simulink model "OMSv1_4"  (Simulink 7.0)
settings: Solver=ode4  SolverMode=SingleTasking  StartTime=0.0  StopTime=4  FixedStep=0.001  MaxStep=0.001  RelTol=1e-3  AbsTol=1e-3
undefined symbols (not defined in the file): alexlaw, bs_onoff, bs_scale, bsfsacrit, bsfsvcrit, cnsgain, fs_onoff, fs_scale, fsdelaycalc, ltdrk, mdlparamlist, phasicgain, pmcgain, pmctau2, pmctau3, saccsw, spgain, tonicgain, tvrD, tvrN
(part 5 of 10)

== system OMSv1_4/OMS v1.4  12/31/07/IM CN-LMLN/BS/FS Logic/BS Enable1/BS Timing ==
  note: (FF init state: Q=0)
  note: * Leading Edge of input ENABLEs output
  note: Operation:
  note: *BS Enabling is initially DISABLED
  note: * Output of TIMER circuit DISABLES output
  note: BS Timing
  From  <= [cmpr] : Inport  OutDataType=sfix(16)  OutScaling=2^0
  timer dur : Inport  Orientation=up  Port=2  OutDataType=sfix(16)  OutScaling=2^0
  Latch1 : Subsystem  mask(Latch){@1=0}
      mask prompts: @1 "Initial State for Output "Q":"
      mask help: Latch
      mask init:
      | ini=(@1~=0);
      mask Help: Latches the S input.  When S (set) is one, the Q output  becomes one.  The output remains one until the R (reset) input becomes one, forcing the output to zero.  If both R and S are one, the latch will be in an undefined state.
      mask Display: disp('S   Q\n\nR  !Q')
  Terminator : Terminator
  event timer2 : Subsystem
      mask Display: disp('Event\nTimer2')
  leading edge detect : Subsystem
      mask Display: disp('Leading\nEdge Det')
  "[bsenab]" : Outport  OutDataType=sfix(16)  OutScaling=2^0  InitialOutput=0
  wires:
  From  <= [cmpr]/1 -> leading edge detect/1(in_1), event timer2/1(_PG)
  leading edge detect/1(out_1) -> Latch1/1(in_1)
  event timer2/1(out_1) -> Latch1/2(in_2)
  Latch1/1(out_1) -> "[bsenab]"/1
  timer dur/1 -> event timer2/2(_timer value (port))
  Latch1/2(out_2) -> Terminator/1

== system OMSv1_4/OMS v1.4  12/31/07/IM CN-LMLN/BS/FS Logic/FS Enable/FS Timing ==
  note: FS Timing
  note: * Output of TIMER circuit DISABLES output
  note: *FS Enabling is initially DISABLED
  note: Operation:
  note: * Leading Edge of input ENABLEs output
  note: (FF init state: Q=0)
  From  <= [cmpr] : Inport  OutDataType=sfix(16)  OutScaling=2^0
  timer dur : Inport  Orientation=up  Port=2  OutDataType=sfix(16)  OutScaling=2^0
  Latch1 : Subsystem  mask(Latch){@1=0}
      mask prompts: @1 "Initial State for Output "Q":"
      mask help: Latch
      mask init:
      | ini=(@1~=0);
      mask Help: Latches the S input.  When S (set) is one, the Q output  becomes one.  The output remains one until the R (reset) input becomes one, forcing the output to zero.  If both R and S are one, the latch will be in an undefined state.
      mask Display: disp('S   Q\n\nR  !Q')
  Terminator : Terminator
  event timer2 : Subsystem
      mask Display: disp('Event\nTimer2')
  leading edge detect : Subsystem
      mask Display: disp('Leading\nEdge Det')
  "[fsenab]" : Outport  OutDataType=sfix(16)  OutScaling=2^0  InitialOutput=0
  wires:
  timer dur/1 -> event timer2/2(_timer value (port))
  Latch1/1(out_1) -> "[fsenab]"/1
  event timer2/1(out_1) -> Latch1/2(in_2)
  leading edge detect/1(out_1) -> Latch1/1(in_1)
  From  <= [cmpr]/1 -> event timer2/1(_PG), leading edge detect/1(in_1)
  Latch1/2(out_2) -> Terminator/1

== system OMSv1_4/OMS v1.4  12/31/07/IM CN-LMLN/BS/FS Logic/FS Enable/SampHold?1 ==
  note: When "S/H?" is LOW, then "Input" is switched directly to the
      | output ("sample").  When "S/H?" is HIGH, the current output is
      | maintained ("hold").
  Input : Inport  OutDataType=sfix(16)  OutScaling=2^0
  S/H? : Inport  Port=2  OutDataType=sfix(16)  OutScaling=2^0
  Memory : Memory  Orientation=left
  Sign : Subsystem
      mask Type: Sign
      mask Description: y = sign(x)
      mask Help: Sign Function:\n\t\t\ty = 1 if x > 0\n\t\t\ty = 0 if x = 0\n\t\t\ty = -1 if x < 0
      mask Display: plot(-50,-50,50,50,[-50,50],[0,0],[0,0],[-50,50],[-40,0],[-30,-30],[0,40],[30,30])
  Switch2 : Switch  Threshold=0.5  SaturateOnIntegerOverflow=on  InputSameDT=on
  output : Outport  OutDataType=sfix(16)  OutScaling=2^0  InitialOutput=0
  wires:
  Input/1 -> Switch2/3
  Memory/1 -> Switch2/1
  S/H?/1 -> Sign/1(in_1)
  Sign/1(out_1) -> Switch2/2
  Switch2/1 -> output/1, Memory/1

== system OMSv1_4/OMS v1.4  12/31/07/IM CN-LMLN/BS/FS Logic/FS Enable/prolong ==
  note: init = 0
  note: init = 0
  note: 11/22/99
  note: The start of the input pulse causes the value on input 1 to be held starting when the leading
      | edge occurs, and this value remains latched until 'delay' seconds after the pulse ends (trailing edge).
  note: The one integration step delay before the S&H block's S/H (bottom) input insures
      | that the input value to be latched is available to theS&H block's top input
      | before the S&H block tries to 'hold'.
  note: Stretch the duration of an input pulse, latching it at its value at pulse onset.
  note: init Q = 0
  value(in) : Inport  OutDataType=sfix(16)  OutScaling=2^0
  " x/1000" : Constant  Orientation=up  Value=0.001  OutDataType=sfix(16)  OutScaling=2^0
  Latch1 : Subsystem  mask(Latch){@1=0}
      mask prompts: @1 "Initial State for Output "Q":"
      mask help: Latch
      mask init:
      | ini=(@1~=0);
      mask Help: Latches the S input.  When S (set) is one, the Q output  becomes one.  The output remains one until the R (reset) input becomes one, forcing the output to zero.  If both R and S are one, the latch will be in an undefined state.
      mask Display: disp('S   Q\n\nR  !Q')
  Product : Product  OutDataType=sfix(16)  OutScaling=2^0  SaturateOnIntegerOverflow=on  RndMeth=Zero  InputSameDT=on
  SampHold?2 : Subsystem
      mask Display: disp('S=L\nH=H')
  Terminator : Terminator
      settings: Orientation=down
  Variable Transport Delay : VariableTransportDelay  MaximumDelay=10  MaximumPoints=prolong_buffersize
  leading edge detect : Subsystem
      mask Display: disp('Leading\nEdge Det')
  loop breaker2 : Memory
  stretch : Constant  Value=prolong  OutDataType=sfix(16)  OutScaling=2^0
  trailing edge detect : Subsystem
      mask Display: disp('Trailing\nEdge Det')
  value(out) : Outport  OutDataType=sfix(16)  OutScaling=2^0  InitialOutput=0
  wires:
  " x/1000"/1 -> Product/2
  Product/1 -> Variable Transport Delay/2
  stretch/1 -> Product/1
  loop breaker2/1 -> SampHold?2/2(S/H?)
  SampHold?2/1(output) -> value(out)/1
  Latch1/1(out_1) -> loop breaker2/1
  leading edge detect/1(out_1) -> Latch1/1(in_1)
  trailing edge detect/1(out_1) -> Variable Transport Delay/1
  Variable Transport Delay/1 -> Latch1/2(in_2)
  value(in)/1 -> SampHold?2/1(Input), trailing edge detect/1(in_1), leading edge detect/1(in_1)
  Latch1/2(out_2) -> Terminator/1

== system OMSv1_4/OMS v1.4  12/31/07/IM CN-LMLN/BS/FS Logic/FS or BS?/Boolify ==
  In1 : Inport  OutDataType=sfix(16)  OutScaling=2^0
  Abs2 : Abs  SaturateOnIntegerOverflow=on
  direction1 : Subsystem
      mask Type: Sign
      mask Description: y = sign(x)
      mask Help: Sign Function:\n\t\t\ty = 1 if x > 0\n\t\t\ty = 0 if x = 0\n\t\t\ty = -1 if x < 0
      mask Display: plot(-50,-50,50,50,[-50,50],[0,0],[0,0],[-50,50],[-40,0],[-30,-30],[0,40],[30,30])
  Out1 : Outport  OutDataType=sfix(16)  OutScaling=2^0  InitialOutput=0
  wires:
  Abs2/1 -> direction1/1(in_1)
  In1/1 -> Abs2/1
  direction1/1(out_1) -> Out1/1

== system OMSv1_4/OMS v1.4  12/31/07/IM CN-LMLN/BS/FS Logic/FS or BS?/SampHold?1 ==
  note: When "S/H?" is LOW, then "Input" is switched directly to the
      | output ("sample").  When "S/H?" is HIGH, the current output is
      | maintained ("hold").
  Input : Inport  OutDataType=sfix(16)  OutScaling=2^0
  S/H? : Inport  Port=2  OutDataType=sfix(16)  OutScaling=2^0
  Memory : Memory  Orientation=left
  Sign : Subsystem
      mask Type: Sign
      mask Description: y = sign(x)
      mask Help: Sign Function:\n\t\t\ty = 1 if x > 0\n\t\t\ty = 0 if x = 0\n\t\t\ty = -1 if x < 0
      mask Display: plot(-50,-50,50,50,[-50,50],[0,0],[0,0],[-50,50],[-40,0],[-30,-30],[0,40],[30,30])
  Switch2 : Switch  Threshold=0.5  SaturateOnIntegerOverflow=on  InputSameDT=on
  output : Outport  OutDataType=sfix(16)  OutScaling=2^0  InitialOutput=0
  wires:
  Input/1 -> Switch2/3
  Memory/1 -> Switch2/1
  S/H?/1 -> Sign/1(in_1)
  Sign/1(out_1) -> Switch2/2
  Switch2/1 -> output/1, Memory/1

== system OMSv1_4/OMS v1.4  12/31/07/IM CN-LMLN/BS/FS Logic/TCHNG Override/Latch1 ==
  in_1 : Inport  OutDataType=sfix(16)  OutScaling=2^0
  in_2 : Inport  Port=2  OutDataType=sfix(16)  OutScaling=2^0
  Demux : Demux  Outputs=2
  Logic : CombinatorialLogic  TruthTable=[0 1;0 1;1 0;0 1;1 0;0 1;1 0;1 0]
  Memory : Memory  Orientation=left  X0=ini
  Mux : Mux  Inputs=3
  out_1 : Outport  OutDataType=sfix(16)  OutScaling=2^0  InitialOutput=0
  out_2 : Outport  Port=2  OutDataType=sfix(16)  OutScaling=2^0  InitialOutput=0
  wires:
  in_2/1 -> Mux/3
  in_1/1 -> Mux/2
  Memory/1 -> Mux/1
  Demux/1 -> Memory/1, out_1/1
  Mux/1 -> Logic/1
  Logic/1 -> Demux/1
  Demux/2 -> out_2/1

== system OMSv1_4/OMS v1.4  12/31/07/IM CN-LMLN/BS/FS Logic/TCHNG Override/event timer2 ==
  note: In 2) Subsequent events DO NOT reset the counter; it only resets when it
      | reaches zero
  note: 2) A new event (leading or trailing edge) is detected. -- Only case 1)
  note: 1) The count reaches its limit (set in "timer value") -- Both case 1) and 2)
  note: In 1), Any event (leading or trailing edge) will reset the counter so that it
      | counts down from the end trailing edge) of that event.
  note: It has TWO modes: 1) Event resettable and 2) Event Non-resettable
  note: The real trick here is understanding how to reload the countdown.
      | It resets if either of two conditions is met:
  note: The "OR" gate allows either of these conditions to reset the circuit.  The delay before the
      | "S" input of the flip-flop prevents both "S" and "R" from being set simultaneously, because
      | this would put the flip-flop in an undefined state.
  note: Therefore, an event first RESETS and then SETS the flip-flop.
  note: (Init input: 0)
  note: (FF init state: Q=0)
  note: (Init input: 0)
  note: This block is an RESETTABLE EVENT TIMER.  It outputs a spike of unit height xx milliseconds
      | (set by "timer value") after it detects an event ( i.e a TRAILING edge which represents the end of a
      |  saccadic pulse)
  note: Resettable
      | Event Timer
  _PG : Inport  OutDataType=sfix(16)  OutScaling=2^0
  _timer value (port) : Inport  Port=2  OutDataType=sfix(16)  OutScaling=2^0
  1 msec : TransportDelay  DelayTime=.001
  Clock : Clock
      settings: Decimation=10
  Latch1 : Subsystem  mask(Latch){@1=0}
      mask prompts: @1 "Initial State for Output "Q":"
      mask help: Latch
      mask init:
      | ini=(@1~=0);
      mask Help: Latches the S input.  When S (set) is one, the Q output  becomes one.  The output remains one until the R (reset) input becomes one, forcing the output to zero.  If both R and S are one, the latch will be in an undefined state.
      mask Display: disp('S   Q\n\nR  !Q')
  Logical Operator : Logic  Operator=OR  Inputs=3
  Logical Operator1 : Logic
  Logical Operator2 : Logic
  Relational Operator : RelationalOperator  InputSameDT=on
  SampHold?1 : Subsystem
      mask Display: disp('S&H\n(S=L)\n(H=H)')
  Sum : Sum  Inputs=+-  OutDataType=sfix(16)  OutScaling=2^0  SaturateOnIntegerOverflow=on  InputSameDT=on
  Terminator : Terminator
  event resettable? : Constant  Orientation=up  Value=0  OutDataType=sfix(16)  OutScaling=2^0
  leading edge detect : Subsystem
      mask Display: disp('Leading\nEdge Det')
  loop breaker : Memory  Orientation=left
  trailing edge detect : Subsystem
      mask Display: disp('Trailing\nEdge Det')
  out_1 : Outport  OutDataType=sfix(16)  OutScaling=2^0  InitialOutput=0
  wires:
  event resettable?/1 -> Logical Operator2/2, Logical Operator1/2
  leading edge detect/1(out_1) -> Logical Operator2/1
  Logical Operator2/1 -> Logical Operator/2
  trailing edge detect/1(out_1) -> Logical Operator1/1, 1 msec/1
  Logical Operator1/1 -> Logical Operator/1
  loop breaker/1 -> Logical Operator/3
  _PG/1 -> leading edge detect/1(in_1), trailing edge detect/1(in_1)
  Latch1/1(out_1) -> SampHold?1/2(S/H?)
  Relational Operator/1 -> out_1/1, loop breaker/1
  Sum/1 -> Relational Operator/1
  Clock/1 -> Sum/1, SampHold?1/1(Input)
  SampHold?1/1(output) -> Sum/2
  Logical Operator/1 -> Latch1/2(in_2)
  1 msec/1 -> Latch1/1(in_1)
  _timer value (port)/1 -> Relational Operator/2
  Latch1/2(out_2) -> Terminator/1

== system OMSv1_4/OMS v1.4  12/31/07/IM CN-LMLN/BS/FS Logic/TCHNG Override/leading edge detect ==
  note: leading edge detection
  in_1 : Inport  OutDataType=sfix(16)  OutScaling=2^0
  Abs : Abs  SaturateOnIntegerOverflow=on
  Derivative : Derivative
  Relational Operator : RelationalOperator  Operator===  InputSameDT=on
  Sign : Subsystem
      mask Type: Sign
      mask Description: y = sign(x)
      mask Help: Sign Function:\n\t\t\ty = 1 if x > 0\n\t\t\ty = 0 if x = 0\n\t\t\ty = -1 if x < 0
      mask Display: plot(-50,-50,50,50,[-50,50],[0,0],[0,0],[-50,50],[-40,0],[-30,-30],[0,40],[30,30])
  Threshold 1 : Constant  OutDataType=sfix(16)  OutScaling=2^0
  out_1 : Outport  OutDataType=sfix(16)  OutScaling=2^0  InitialOutput=0
  wires:
  in_1/1 -> Abs/1
  Relational Operator/1 -> out_1/1
  Threshold 1/1 -> Relational Operator/2
  Sign/1(out_1) -> Relational Operator/1
  Derivative/1 -> Sign/1(in_1)
  Abs/1 -> Derivative/1

== system OMSv1_4/OMS v1.4  12/31/07/IM CN-LMLN/BS/FS Logic/prolong/Latch1 ==
  in_1 : Inport  OutDataType=sfix(16)  OutScaling=2^0
  in_2 : Inport  Port=2  OutDataType=sfix(16)  OutScaling=2^0
  Demux : Demux  Outputs=2
  Logic : CombinatorialLogic  TruthTable=[0 1;0 1;1 0;0 1;1 0;0 1;1 0;1 0]
  Memory : Memory  Orientation=left  X0=ini
  Mux : Mux  Inputs=3
  out_1 : Outport  OutDataType=sfix(16)  OutScaling=2^0  InitialOutput=0
  out_2 : Outport  Port=2  OutDataType=sfix(16)  OutScaling=2^0  InitialOutput=0
  wires:
  in_2/1 -> Mux/3
  in_1/1 -> Mux/2
  Memory/1 -> Mux/1
  Demux/1 -> Memory/1, out_1/1
  Mux/1 -> Logic/1
  Logic/1 -> Demux/1
  Demux/2 -> out_2/1

== system OMSv1_4/OMS v1.4  12/31/07/IM CN-LMLN/BS/FS Logic/prolong/SampHold?2 ==
  note: When "S/H?" is LOW, then "Input" is switched directly to the
      | output ("sample").  When "S/H?" is HIGH, the current output is
      | maintained ("hold").
  Input : Inport  OutDataType=sfix(16)  OutScaling=2^0
  S/H? : Inport  Port=2  OutDataType=sfix(16)  OutScaling=2^0
  Memory : Memory  Orientation=left
  Sign : Subsystem
      mask Type: Sign
      mask Description: y = sign(x)
      mask Help: Sign Function:\n\t\t\ty = 1 if x > 0\n\t\t\ty = 0 if x = 0\n\t\t\ty = -1 if x < 0
      mask Display: plot(-50,-50,50,50,[-50,50],[0,0],[0,0],[-50,50],[-40,0],[-30,-30],[0,40],[30,30])
  Switch2 : Switch  Threshold=0.5  SaturateOnIntegerOverflow=on  InputSameDT=on
  output : Outport  OutDataType=sfix(16)  OutScaling=2^0  InitialOutput=0
  wires:
  S/H?/1 -> Sign/1(in_1)
  Sign/1(out_1) -> Switch2/2
  Input/1 -> Switch2/3
  Switch2/1 -> Memory/1, output/1
  Memory/1 -> Switch2/1

== system OMSv1_4/OMS v1.4  12/31/07/IM CN-LMLN/BS/FS Logic/prolong/leading edge detect ==
  note: leading edge detection
  in_1 : Inport  OutDataType=sfix(16)  OutScaling=2^0
  Abs : Abs  SaturateOnIntegerOverflow=on
  Derivative : Derivative
  Relational Operator : RelationalOperator  Operator===  InputSameDT=on
  Sign : Subsystem
      mask Type: Sign
      mask Description: y = sign(x)
      mask Help: Sign Function:\n\t\t\ty = 1 if x > 0\n\t\t\ty = 0 if x = 0\n\t\t\ty = -1 if x < 0
      mask Display: plot(-50,-50,50,50,[-50,50],[0,0],[0,0],[-50,50],[-40,0],[-30,-30],[0,40],[30,30])
  Threshold 1 : Constant  OutDataType=sfix(16)  OutScaling=2^0
  out_1 : Outport  OutDataType=sfix(16)  OutScaling=2^0  InitialOutput=0
  wires:
  in_1/1 -> Abs/1
  Relational Operator/1 -> out_1/1
  Threshold 1/1 -> Relational Operator/2
  Sign/1(out_1) -> Relational Operator/1
  Derivative/1 -> Sign/1(in_1)
  Abs/1 -> Derivative/1

== system OMSv1_4/OMS v1.4  12/31/07/IM CN-LMLN/BS/FS Logic/prolong/trailing edge detect ==
  note: It is also possible to remove the SIGNUM function
      | and the '==', and replace them with a simple
      | switch with a threshold of (say) 150 or so.
  note: trailing edge detection
  in_1 : Inport  OutDataType=sfix(16)  OutScaling=2^0
  Abs : Abs  SaturateOnIntegerOverflow=on
  Derivative : Derivative
  Relational Operator : RelationalOperator  Operator===  InputSameDT=on
  Sign : Subsystem
      mask Type: Sign
      mask Description: y = sign(x)
      mask Help: Sign Function:\n\t\t\ty = 1 if x > 0\n\t\t\ty = 0 if x = 0\n\t\t\ty = -1 if x < 0
      mask Display: plot(-50,-50,50,50,[-50,50],[0,0],[0,0],[-50,50],[-40,0],[-30,-30],[0,40],[30,30])
  Threshold 1 : Constant  Value=-1  OutDataType=sfix(16)  OutScaling=2^0
  out_1 : Outport  OutDataType=sfix(16)  OutScaling=2^0  InitialOutput=0
  wires:
  Abs/1 -> Derivative/1
  Derivative/1 -> Sign/1(in_1)
  Sign/1(out_1) -> Relational Operator/1
  Threshold 1/1 -> Relational Operator/2
  Relational Operator/1 -> out_1/1
  in_1/1 -> Abs/1

== system OMSv1_4/OMS v1.4  12/31/07/IM CN-LMLN/MdlPlnt+2/OMN3/SampHold? ==
  note: When "S/H?" is LOW, then "Input" is switched directly to the
      | output ("sample").  When "S/H?" is HIGH, the current output is
      | maintained ("hold").
  Input : Inport  OutDataType=sfix(16)  OutScaling=2^0
  S/H? : Inport  Port=2  OutDataType=sfix(16)  OutScaling=2^0
  Memory : Memory  Orientation=left
  Sign : Subsystem
      mask Type: Sign
      mask Description: y = sign(x)
      mask Help: Sign Function:\n\t\t\ty = 1 if x > 0\n\t\t\ty = 0 if x = 0\n\t\t\ty = -1 if x < 0
      mask Display: plot(-50,-50,50,50,[-50,50],[0,0],[0,0],[-50,50],[-40,0],[-30,-30],[0,40],[30,30])
  Switch2 : Switch  Threshold=0.5  SaturateOnIntegerOverflow=on  InputSameDT=on
  output : Outport  OutDataType=sfix(16)  OutScaling=2^0  InitialOutput=0
  wires:
  Switch2/1 -> Memory/1, output/1
  Memory/1 -> Switch2/1
  Input/1 -> Switch2/3
  Sign/1(out_1) -> Switch2/2
  S/H?/1 -> Sign/1(in_1)

== system OMSv1_4/OMS v1.4  12/31/07/IM CN-LMLN/MdlPlnt+2/OMN3/Sign ==
  in_1 : Inport  OutDataType=sfix(16)  OutScaling=2^0
  Constant : Constant  Value=0  OutDataType=sfix(16)  OutScaling=2^0
  Relational Operator : RelationalOperator  Operator=>  InputSameDT=on
  Relational Operator1 : RelationalOperator  Operator=<  InputSameDT=on
  Sum : Sum  Inputs=+-  OutDataType=sfix(16)  OutScaling=2^0  SaturateOnIntegerOverflow=on  InputSameDT=on
  out_1 : Outport  OutDataType=sfix(16)  OutScaling=2^0  InitialOutput=0
  wires:
  Sum/1 -> out_1/1
  Relational Operator/1 -> Sum/1
  Relational Operator1/1 -> Sum/2
  Constant/1 -> Relational Operator1/2, Relational Operator/2
  in_1/1 -> Relational Operator/1, Relational Operator1/1

== system OMSv1_4/OMS v1.4  12/31/07/IM CN-LMLN/NI Control/Boolify/direction1 ==
  in_1 : Inport  OutDataType=sfix(16)  OutScaling=2^0
  Constant : Constant  Value=0  OutDataType=sfix(16)  OutScaling=2^0
  Relational Operator : RelationalOperator  Operator=>  InputSameDT=on
  Relational Operator1 : RelationalOperator  Operator=<  InputSameDT=on
  Sum : Sum  Inputs=+-  OutDataType=sfix(16)  OutScaling=2^0  SaturateOnIntegerOverflow=on  InputSameDT=on
  out_1 : Outport  OutDataType=sfix(16)  OutScaling=2^0  InitialOutput=0
  wires:
  in_1/1 -> Relational Operator/1, Relational Operator1/1
  Constant/1 -> Relational Operator1/2, Relational Operator/2
  Relational Operator1/1 -> Sum/2
  Relational Operator/1 -> Sum/1
  Sum/1 -> out_1/1

== system OMSv1_4/OMS v1.4  12/31/07/IM CN-LMLN/NI Control/Boolify1/direction1 ==
  in_1 : Inport  OutDataType=sfix(16)  OutScaling=2^0
  Constant : Constant  Value=0  OutDataType=sfix(16)  OutScaling=2^0
  Relational Operator : RelationalOperator  Operator=>  InputSameDT=on
  Relational Operator1 : RelationalOperator  Operator=<  InputSameDT=on
  Sum : Sum  Inputs=+-  OutDataType=sfix(16)  OutScaling=2^0  SaturateOnIntegerOverflow=on  InputSameDT=on
  out_1 : Outport  OutDataType=sfix(16)  OutScaling=2^0  InitialOutput=0
  wires:
  Sum/1 -> out_1/1
  Relational Operator/1 -> Sum/1
  Relational Operator1/1 -> Sum/2
  Constant/1 -> Relational Operator/2, Relational Operator1/2
  in_1/1 -> Relational Operator1/1, Relational Operator/1

== system OMSv1_4/OMS v1.4  12/31/07/IM CN-LMLN/NI Control/Boolify2/direction1 ==
  in_1 : Inport  OutDataType=sfix(16)  OutScaling=2^0
  Constant : Constant  Value=0  OutDataType=sfix(16)  OutScaling=2^0
  Relational Operator : RelationalOperator  Operator=>  InputSameDT=on
  Relational Operator1 : RelationalOperator  Operator=<  InputSameDT=on
  Sum : Sum  Inputs=+-  OutDataType=sfix(16)  OutScaling=2^0  SaturateOnIntegerOverflow=on  InputSameDT=on
  out_1 : Outport  OutDataType=sfix(16)  OutScaling=2^0  InitialOutput=0
  wires:
  in_1/1 -> Relational Operator/1, Relational Operator1/1
  Constant/1 -> Relational Operator1/2, Relational Operator/2
  Relational Operator1/1 -> Sum/2
  Relational Operator/1 -> Sum/1
  Sum/1 -> out_1/1

== system OMSv1_4/OMS v1.4  12/31/07/IM CN-LMLN/NI Control/Boolify3/direction1 ==
  in_1 : Inport  OutDataType=sfix(16)  OutScaling=2^0
  Constant : Constant  Value=0  OutDataType=sfix(16)  OutScaling=2^0
  Relational Operator : RelationalOperator  Operator=>  InputSameDT=on
  Relational Operator1 : RelationalOperator  Operator=<  InputSameDT=on
  Sum : Sum  Inputs=+-  OutDataType=sfix(16)  OutScaling=2^0  SaturateOnIntegerOverflow=on  InputSameDT=on
  out_1 : Outport  OutDataType=sfix(16)  OutScaling=2^0  InitialOutput=0
  wires:
  Sum/1 -> out_1/1
  Relational Operator/1 -> Sum/1
  Relational Operator1/1 -> Sum/2
  Constant/1 -> Relational Operator/2, Relational Operator1/2
  in_1/1 -> Relational Operator1/1, Relational Operator/1

== system OMSv1_4/OMS v1.4  12/31/07/IM CN-LMLN/NI Control/Zero-Cross/Sign2 ==
  in_1 : Inport  OutDataType=sfix(16)  OutScaling=2^0
  Constant : Constant  Value=0  OutDataType=sfix(16)  OutScaling=2^0
  Relational Operator : RelationalOperator  Operator=>  InputSameDT=on
  Relational Operator1 : RelationalOperator  Operator=<  InputSameDT=on
  Sum : Sum  Inputs=+-  OutDataType=sfix(16)  OutScaling=2^0  SaturateOnIntegerOverflow=on  InputSameDT=on
  out_1 : Outport  OutDataType=sfix(16)  OutScaling=2^0  InitialOutput=0
  wires:
  in_1/1 -> Relational Operator/1, Relational Operator1/1
  Constant/1 -> Relational Operator1/2, Relational Operator/2
  Relational Operator1/1 -> Sum/2
  Relational Operator/1 -> Sum/1
  Sum/1 -> out_1/1

== system OMSv1_4/OMS v1.4  12/31/07/IM CN-LMLN/NI Control/leading edge detect/Sign ==
  in_1 : Inport  OutDataType=sfix(16)  OutScaling=2^0
  Constant : Constant  Value=0  OutDataType=sfix(16)  OutScaling=2^0
  Relational Operator : RelationalOperator  Operator=>  InputSameDT=on
  Relational Operator1 : RelationalOperator  Operator=<  InputSameDT=on
  Sum : Sum  Inputs=+-  OutDataType=sfix(16)  OutScaling=2^0  SaturateOnIntegerOverflow=on  InputSameDT=on
  out_1 : Outport  OutDataType=sfix(16)  OutScaling=2^0  InitialOutput=0
  wires:
  Sum/1 -> out_1/1
  Relational Operator/1 -> Sum/1
  Relational Operator1/1 -> Sum/2
  Constant/1 -> Relational Operator1/2, Relational Operator/2
  in_1/1 -> Relational Operator/1, Relational Operator1/1

== system OMSv1_4/OMS v1.4  12/31/07/IM CN-LMLN/NI Control/leading edge detect1/Sign ==
  in_1 : Inport  OutDataType=sfix(16)  OutScaling=2^0
  Constant : Constant  Value=0  OutDataType=sfix(16)  OutScaling=2^0
  Relational Operator : RelationalOperator  Operator=>  InputSameDT=on
  Relational Operator1 : RelationalOperator  Operator=<  InputSameDT=on
  Sum : Sum  Inputs=+-  OutDataType=sfix(16)  OutScaling=2^0  SaturateOnIntegerOverflow=on  InputSameDT=on
  out_1 : Outport  OutDataType=sfix(16)  OutScaling=2^0  InitialOutput=0
  wires:
  in_1/1 -> Relational Operator1/1, Relational Operator/1
  Constant/1 -> Relational Operator/2, Relational Operator1/2
  Relational Operator1/1 -> Sum/2
  Relational Operator/1 -> Sum/1
  Sum/1 -> out_1/1

== system OMSv1_4/OMS v1.4  12/31/07/IM CN-LMLN/NI Control/trailing edge detect/Sign ==
  in_1 : Inport  OutDataType=sfix(16)  OutScaling=2^0
  Constant : Constant  Value=0  OutDataType=sfix(16)  OutScaling=2^0
  Relational Operator : RelationalOperator  Operator=>  InputSameDT=on
  Relational Operator1 : RelationalOperator  Operator=<  InputSameDT=on
  Sum : Sum  Inputs=+-  OutDataType=sfix(16)  OutScaling=2^0  SaturateOnIntegerOverflow=on  InputSameDT=on
  out_1 : Outport  OutDataType=sfix(16)  OutScaling=2^0  InitialOutput=0
  wires:
  in_1/1 -> Relational Operator/1, Relational Operator1/1
  Constant/1 -> Relational Operator1/2, Relational Operator/2
  Relational Operator1/1 -> Sum/2
  Relational Operator/1 -> Sum/1
  Sum/1 -> out_1/1

== system OMSv1_4/OMS v1.4  12/31/07/IM CN-LMLN/Sacc Blank/event timer1/Latch1 ==
  in_1 : Inport  OutDataType=sfix(16)  OutScaling=2^0
  in_2 : Inport  Port=2  OutDataType=sfix(16)  OutScaling=2^0
  Demux : Demux  Outputs=2
  Logic : CombinatorialLogic  TruthTable=[0 1;0 1;1 0;0 1;1 0;0 1;1 0;1 0]
  Memory : Memory  Orientation=left  X0=ini
  Mux : Mux  Inputs=3
  out_1 : Outport  OutDataType=sfix(16)  OutScaling=2^0  InitialOutput=0
  out_2 : Outport  Port=2  OutDataType=sfix(16)  OutScaling=2^0  InitialOutput=0
  wires:
  in_2/1 -> Mux/3
  in_1/1 -> Mux/2
  Memory/1 -> Mux/1
  Demux/1 -> out_1/1, Memory/1
  Mux/1 -> Logic/1
  Logic/1 -> Demux/1
  Demux/2 -> out_2/1

== system OMSv1_4/OMS v1.4  12/31/07/IM CN-LMLN/Sacc Blank/event timer1/SampHold?1 ==
  note: When "S/H?" is LOW, then "Input" is switched directly to the
      | output ("sample").  When "S/H?" is HIGH, the current output is
      | maintained ("hold").
  Input : Inport  OutDataType=sfix(16)  OutScaling=2^0
  S/H? : Inport  Port=2  OutDataType=sfix(16)  OutScaling=2^0
  Memory : Memory  Orientation=left
  Sign : Subsystem
      mask Type: Sign
      mask Description: y = sign(x)
      mask Help: Sign Function:\n\t\t\ty = 1 if x > 0\n\t\t\ty = 0 if x = 0\n\t\t\ty = -1 if x < 0
      mask Display: plot(-50,-50,50,50,[-50,50],[0,0],[0,0],[-50,50],[-40,0],[-30,-30],[0,40],[30,30])
  Switch2 : Switch  Threshold=0.5  SaturateOnIntegerOverflow=on  InputSameDT=on
  output : Outport  OutDataType=sfix(16)  OutScaling=2^0  InitialOutput=0
  wires:
  Switch2/1 -> Memory/1, output/1
  Sign/1(out_1) -> Switch2/2
  S/H?/1 -> Sign/1(in_1)
  Memory/1 -> Switch2/1
  Input/1 -> Switch2/3

== system OMSv1_4/OMS v1.4  12/31/07/IM CN-LMLN/Sacc Blank/event timer1/leading edge detect ==
  note: It is also possible to remove the SIGNUM function
      | and the '==', and replace them with a simple
      | switch with a threshold of (say) 150 or so.
  note: leading edge detection
  in_1 : Inport  OutDataType=sfix(16)  OutScaling=2^0
  Abs : Abs  SaturateOnIntegerOverflow=on
  Derivative : Derivative
  Relational Operator : RelationalOperator  Operator===  InputSameDT=on
  Sign : Subsystem
      mask Type: Sign
      mask Description: y = sign(x)
      mask Help: Sign Function:\n\t\t\ty = 1 if x > 0\n\t\t\ty = 0 if x = 0\n\t\t\ty = -1 if x < 0
      mask Display: plot(-50,-50,50,50,[-50,50],[0,0],[0,0],[-50,50],[-40,0],[-30,-30],[0,40],[30,30])
  Threshold 1 : Constant  OutDataType=sfix(16)  OutScaling=2^0
  out_1 : Outport  OutDataType=sfix(16)  OutScaling=2^0  InitialOutput=0
  wires:
  Abs/1 -> Derivative/1
  Derivative/1 -> Sign/1(in_1)
  Sign/1(out_1) -> Relational Operator/1
  Threshold 1/1 -> Relational Operator/2
  Relational Operator/1 -> out_1/1
  in_1/1 -> Abs/1

== system OMSv1_4/OMS v1.4  12/31/07/IM CN-LMLN/Sacc Blank/event timer1/trailing edge detect ==
  note: trailing edge detection
  note: It is also possible to remove the SIGNUM function
      | and the '==', and replace them with a simple
      | switch with a threshold of (say) 150 or so.
  in_1 : Inport  OutDataType=sfix(16)  OutScaling=2^0
  Abs : Abs  SaturateOnIntegerOverflow=on
  Derivative : Derivative
  Relational Operator : RelationalOperator  Operator===  InputSameDT=on
  Sign : Subsystem
      mask Type: Sign
      mask Description: y = sign(x)
      mask Help: Sign Function:\n\t\t\ty = 1 if x > 0\n\t\t\ty = 0 if x = 0\n\t\t\ty = -1 if x < 0
      mask Display: plot(-50,-50,50,50,[-50,50],[0,0],[0,0],[-50,50],[-40,0],[-30,-30],[0,40],[30,30])
  Threshold 1 : Constant  Value=-1  OutDataType=sfix(16)  OutScaling=2^0
  out_1 : Outport  OutDataType=sfix(16)  OutScaling=2^0  InitialOutput=0
  wires:
  in_1/1 -> Abs/1
  Relational Operator/1 -> out_1/1
  Threshold 1/1 -> Relational Operator/2
  Sign/1(out_1) -> Relational Operator/1
  Derivative/1 -> Sign/1(in_1)
  Abs/1 -> Derivative/1

== system OMSv1_4/OMS v1.4  12/31/07/IM CN-LMLN/Sacc Blank/leading edge detect/Sign ==
  in_1 : Inport  OutDataType=sfix(16)  OutScaling=2^0
  Constant : Constant  Value=0  OutDataType=sfix(16)  OutScaling=2^0
  Relational Operator : RelationalOperator  Operator=>  InputSameDT=on
  Relational Operator1 : RelationalOperator  Operator=<  InputSameDT=on
  Sum : Sum  Inputs=+-  OutDataType=sfix(16)  OutScaling=2^0  SaturateOnIntegerOverflow=on  InputSameDT=on
  out_1 : Outport  OutDataType=sfix(16)  OutScaling=2^0  InitialOutput=0
  wires:
  in_1/1 -> Relational Operator/1, Relational Operator1/1
  Constant/1 -> Relational Operator1/2, Relational Operator/2
  Relational Operator1/1 -> Sum/2
  Relational Operator/1 -> Sum/1
  Sum/1 -> out_1/1

== system OMSv1_4/OMS v1.4  12/31/07/IM CN-LMLN/Sacc Blank/rising edge detect/Sign ==
  in_1 : Inport  OutDataType=sfix(16)  OutScaling=2^0
  Constant : Constant  Value=0  OutDataType=sfix(16)  OutScaling=2^0
  Relational Operator : RelationalOperator  Operator=>  InputSameDT=on
  Relational Operator1 : RelationalOperator  Operator=<  InputSameDT=on
  Sum : Sum  Inputs=+-  OutDataType=sfix(16)  OutScaling=2^0  SaturateOnIntegerOverflow=on  InputSameDT=on
  out_1 : Outport  OutDataType=sfix(16)  OutScaling=2^0  InitialOutput=0
  wires:
  in_1/1 -> Relational Operator1/1, Relational Operator/1
  Constant/1 -> Relational Operator/2, Relational Operator1/2
  Relational Operator1/1 -> Sum/2
  Relational Operator/1 -> Sum/1
  Sum/1 -> out_1/1

== system OMSv1_4/OMS v1.4  12/31/07/IM CN-LMLN/Sacc Blank/rising edge detect1/Sign ==
  in_1 : Inport  OutDataType=sfix(16)  OutScaling=2^0
  Constant : Constant  Value=0  OutDataType=sfix(16)  OutScaling=2^0
  Relational Operator : RelationalOperator  Operator=>  InputSameDT=on
  Relational Operator1 : RelationalOperator  Operator=<  InputSameDT=on
  Sum : Sum  Inputs=+-  OutDataType=sfix(16)  OutScaling=2^0  SaturateOnIntegerOverflow=on  InputSameDT=on
  out_1 : Outport  OutDataType=sfix(16)  OutScaling=2^0  InitialOutput=0
  wires:
  Sum/1 -> out_1/1
  Relational Operator/1 -> Sum/1
  Relational Operator1/1 -> Sum/2
  Constant/1 -> Relational Operator/2, Relational Operator1/2
  in_1/1 -> Relational Operator1/1, Relational Operator/1

== system OMSv1_4/OMS v1.4  12/31/07/IM CN-LMLN/Saccade Enable/Enable Control/2 ms ==
  note: init Q = 0
  note: Stretch the duration of an input pulse, latching it at its value at pulse onset.
  note: The one integration step delay before the S&H block's S/H (bottom) input insures
      | that the input value to be latched is available to theS&H block's top input
      | before the S&H block tries to 'hold'.
  note: The start of the input pulse causes the value on input 1 to be held starting when the leading
      | edge occurs, and this value remains latched until 'delay' seconds after the pulse ends (trailing edge).
  note: 11/22/99
  note: init = 0
  note: init = 0
  value(in) : Inport  OutDataType=sfix(16)  OutScaling=2^0
  " x/1000" : Constant  Orientation=up  Value=0.001  OutDataType=sfix(16)  OutScaling=2^0
  Latch1 : Subsystem  mask(Latch){@1=0}
      mask prompts: @1 "Initial State for Output "Q":"
      mask help: Latch
      mask init:
      | ini=(@1~=0);
      mask Help: Latches the S input.  When S (set) is one, the Q output  becomes one.  The output remains one until the R (reset) input becomes one, forcing the output to zero.  If both R and S are one, the latch will be in an undefined state.
      mask Display: disp('S   Q\n\nR  !Q')
  Product : Product  OutDataType=sfix(16)  OutScaling=2^0  SaturateOnIntegerOverflow=on  RndMeth=Zero  InputSameDT=on
  SampHold?2 : Subsystem
      mask Display: disp('S=L\nH=H')
  Terminator : Terminator
  Variable Transport Delay : VariableTransportDelay  MaximumDelay=10  MaximumPoints=prolong_buffersize
  leading edge detect : Subsystem
      mask Display: disp('Leading\nEdge Det')
  loop breaker2 : Memory
  stretch : Constant  Value=prolong  OutDataType=sfix(16)  OutScaling=2^0
  trailing edge detect : Subsystem
      mask Display: disp('Trailing\nEdge Det')
  value(out) : Outport  OutDataType=sfix(16)  OutScaling=2^0  InitialOutput=0
  wires:
  value(in)/1 -> leading edge detect/1(in_1), trailing edge detect/1(in_1), SampHold?2/1(Input)
  Variable Transport Delay/1 -> Latch1/2(in_2)
  trailing edge detect/1(out_1) -> Variable Transport Delay/1
  leading edge detect/1(out_1) -> Latch1/1(in_1)
  Latch1/1(out_1) -> loop breaker2/1
  SampHold?2/1(output) -> value(out)/1
  loop breaker2/1 -> SampHold?2/2(S/H?)
  stretch/1 -> Product/1
  Product/1 -> Variable Transport Delay/2
  " x/1000"/1 -> Product/2
  Latch1/2(out_2) -> Terminator/1

== system OMSv1_4/OMS v1.4  12/31/07/IM CN-LMLN/Saccade Enable/Enable Control/50 ms ==
  note: init = 0
  note: init = 0
  note: 11/22/99
  note: The start of the input pulse causes the value on input 1 to be held starting when the leading
      | edge occurs, and this value remains latched until 'delay' seconds after the pulse ends (trailing edge).
  note: The one integration step delay before the S&H block's S/H (bottom) input insures
      | that the input value to be latched is available to theS&H block's top input
      | before the S&H block tries to 'hold'.
  note: Stretch the duration of an input pulse, latching it at its value at pulse onset.
  note: init Q = 0
  value(in) : Inport  OutDataType=sfix(16)  OutScaling=2^0
  " x/1000" : Constant  Orientation=up  Value=0.001  OutDataType=sfix(16)  OutScaling=2^0
  Latch1 : Subsystem  mask(Latch){@1=0}
      mask prompts: @1 "Initial State for Output "Q":"
      mask help: Latch
      mask init:
      | ini=(@1~=0);
      mask Help: Latches the S input.  When S (set) is one, the Q output  becomes one.  The output remains one until the R (reset) input becomes one, forcing the output to zero.  If both R and S are one, the latch will be in an undefined state.
      mask Display: disp('S   Q\n\nR  !Q')
  Product : Product  OutDataType=sfix(16)  OutScaling=2^0  SaturateOnIntegerOverflow=on  RndMeth=Zero  InputSameDT=on
  SampHold?2 : Subsystem
      mask Display: disp('S=L\nH=H')
  Terminator : Terminator
  Variable Transport Delay : VariableTransportDelay  MaximumDelay=10  MaximumPoints=prolong_buffersize
  leading edge detect : Subsystem
      mask Display: disp('Leading\nEdge Det')
  loop breaker2 : Memory
  stretch : Constant  Value=prolong  OutDataType=sfix(16)  OutScaling=2^0
  trailing edge detect : Subsystem
      mask Display: disp('Trailing\nEdge Det')
  value(out) : Outport  OutDataType=sfix(16)  OutScaling=2^0  InitialOutput=0
  wires:
  " x/1000"/1 -> Product/2
  Product/1 -> Variable Transport Delay/2
  stretch/1 -> Product/1
  loop breaker2/1 -> SampHold?2/2(S/H?)
  SampHold?2/1(output) -> value(out)/1
  Latch1/1(out_1) -> loop breaker2/1
  leading edge detect/1(out_1) -> Latch1/1(in_1)
  trailing edge detect/1(out_1) -> Variable Transport Delay/1
  Variable Transport Delay/1 -> Latch1/2(in_2)
  value(in)/1 -> SampHold?2/1(Input), trailing edge detect/1(in_1), leading edge detect/1(in_1)
  Latch1/2(out_2) -> Terminator/1

== system OMSv1_4/OMS v1.4  12/31/07/IM CN-LMLN/Saccade Enable/Enable Control/Boolify ==
  In1 : Inport  OutDataType=sfix(16)  OutScaling=2^0
  Abs2 : Abs  SaturateOnIntegerOverflow=on
  direction1 : Subsystem
      mask Type: Sign
      mask Description: y = sign(x)
      mask Help: Sign Function:\n\t\t\ty = 1 if x > 0\n\t\t\ty = 0 if x = 0\n\t\t\ty = -1 if x < 0
      mask Display: plot(-50,-50,50,50,[-50,50],[0,0],[0,0],[-50,50],[-40,0],[-30,-30],[0,40],[30,30])
  Out1 : Outport  OutDataType=sfix(16)  OutScaling=2^0  InitialOutput=0
  wires:
  Abs2/1 -> direction1/1(in_1)
  In1/1 -> Abs2/1
  direction1/1(out_1) -> Out1/1

== system OMSv1_4/OMS v1.4  12/31/07/IM CN-LMLN/Saccade Enable/Enable Control/Boolify1 ==
  In1 : Inport  OutDataType=sfix(16)  OutScaling=2^0
  Abs2 : Abs  SaturateOnIntegerOverflow=on
  direction1 : Subsystem
      mask Type: Sign
      mask Description: y = sign(x)
      mask Help: Sign Function:\n\t\t\ty = 1 if x > 0\n\t\t\ty = 0 if x = 0\n\t\t\ty = -1 if x < 0
      mask Display: plot(-50,-50,50,50,[-50,50],[0,0],[0,0],[-50,50],[-40,0],[-30,-30],[0,40],[30,30])
  Out1 : Outport  OutDataType=sfix(16)  OutScaling=2^0  InitialOutput=0
  wires:
  Abs2/1 -> direction1/1(in_1)
  In1/1 -> Abs2/1
  direction1/1(out_1) -> Out1/1

== system OMSv1_4/OMS v1.4  12/31/07/IM CN-LMLN/Saccade Enable/Enable Control/Boolify2 ==
  In1 : Inport  OutDataType=sfix(16)  OutScaling=2^0
  Abs2 : Abs  SaturateOnIntegerOverflow=on
  direction1 : Subsystem
      mask Type: Sign
      mask Description: y = sign(x)
      mask Help: Sign Function:\n\t\t\ty = 1 if x > 0\n\t\t\ty = 0 if x = 0\n\t\t\ty = -1 if x < 0
      mask Display: plot(-50,-50,50,50,[-50,50],[0,0],[0,0],[-50,50],[-40,0],[-30,-30],[0,40],[30,30])
  Out1 : Outport  OutDataType=sfix(16)  OutScaling=2^0  InitialOutput=0
  wires:
  Abs2/1 -> direction1/1(in_1)
  In1/1 -> Abs2/1
  direction1/1(out_1) -> Out1/1

== system OMSv1_4/OMS v1.4  12/31/07/IM CN-LMLN/Saccade Enable/Enable Control/ECPY Timing ==
  note: ECPY Timing
  note: (Init input:0)
  note: (Init input: 1)
  note: (FF init state: Q=0)
  note: (Init input: 0)
  note: (FF init state: Q=0)
  note: (((see original refract latch block for full description of operation.)))
  note: This signal is used by the Internal Monitor to decide when to compare EFERENCE COPY eye position with old eye position to decide if an appropriate saccade was made.
  note: This block outputs an ENABLE signal xx milliseconds long (set in "enable duration"), starting xx milliseconds (set in "post-pulse delay time") AFTER the input pulse concludes.
  note: If the FF init state is 0, then the block's initial output will be zero. If the FF init state is 1, then the block's initial output will be one.
  note: Corrective Saccades
  ECPY EnCntr [ecenctrl] : Inport  OutDataType=sfix(16)  OutScaling=2^0
  Latch2 : Subsystem  mask(Latch){@1=0}
      mask prompts: @1 "Initial State for Output "Q":"
      mask help: Latch
      mask init:
      | ini=(@1~=0);
      mask Help: Latches the S input.  When S (set) is one, the Q output becomes one.  The output remains one until the R (reset) input becomes one, forcing the output to zero.  If both R and S are one, the latch will be in an undefined state.
      mask Display: disp('S   Q\n\nR  !Q')
  Latch4 : Subsystem  mask(Latch){@1=0}
      mask prompts: @1 "Initial State for Output "Q":"
      mask help: Latch
      mask init:
      | ini=(@1~=0);
      mask Help: Latches the S input.  When S (set) is one, the Q output becomes one.  The output remains one until the R (reset) input becomes one, forcing the output to zero.  If both R and S are one, the latch will be in an undefined state.
      mask Display: disp('S   Q\n\nR  !Q')
  Switch1 : Switch  Threshold=.5  SaturateOnIntegerOverflow=on  InputSameDT=on
  Terminator : Terminator
  Threshold 3 : Constant  Orientation=left  Value=0  OutDataType=sfix(16)  OutScaling=2^0
  enab dur 10ms : TransportDelay  DelayTime=.01  InitialOutput=1
  leading edge detect : Subsystem
      mask Display: disp('Leading\nEdge Det')
  leading edge detect1 : Subsystem
      mask Display: disp('Leading\nEdge Det')
  loop breaker : Memory  Orientation=left
  or : Logic  Operator=OR
  post-pulse delay 130ms : TransportDelay  DelayTime=.13
  trailing edge detect : Subsystem
      mask Display: disp('Trailing\nEdge Det')
  ECPY Enable [ecpyenab] : Outport  OutDataType=sfix(16)  OutScaling=2^0  InitialOutput=0
  wires:
  or/1 -> Latch4/2(in_2)
  trailing edge detect/1(out_1) -> or/1, post-pulse delay 130ms/1
  Switch1/1 -> leading edge detect1/1(in_1), trailing edge detect/1(in_1)
  leading edge detect1/1(out_1) -> or/2
  ECPY EnCntr [ecenctrl]/1 -> Switch1/1
  Threshold 3/1 -> Switch1/3
  loop breaker/1 -> Switch1/2
  Latch2/1(out_1) -> ECPY Enable [ecpyenab]/1
  leading edge detect/1(out_1) -> enab dur 10ms/1, Latch2/1(in_1)
  enab dur 10ms/1 -> Latch2/2(in_2)
  Latch2/2(out_2) -> loop breaker/1
  post-pulse delay 130ms/1 -> Latch4/1(in_1)
  Latch4/1(out_1) -> leading edge detect/1(in_1)
  Latch4/2(out_2) -> Terminator/1

== system OMSv1_4/OMS v1.4  12/31/07/IM CN-LMLN/Saccade Enable/Enable Control/Latch1 ==
  in_1 : Inport  OutDataType=sfix(16)  OutScaling=2^0
  in_2 : Inport  Port=2  OutDataType=sfix(16)  OutScaling=2^0
  Demux : Demux  Outputs=2
  Logic : CombinatorialLogic  TruthTable=[0 1;0 1;1 0;0 1;1 0;0 1;1 0;1 0]
  Memory : Memory  Orientation=left  X0=ini
  Mux : Mux  Inputs=3
  out_1 : Outport  OutDataType=sfix(16)  OutScaling=2^0  InitialOutput=0
  out_2 : Outport  Port=2  OutDataType=sfix(16)  OutScaling=2^0  InitialOutput=0
  wires:
  Demux/2 -> out_2/1
  Logic/1 -> Demux/1
  Mux/1 -> Logic/1
  Demux/1 -> out_1/1, Memory/1
  Memory/1 -> Mux/1
  in_1/1 -> Mux/2
  in_2/1 -> Mux/3

== system OMSv1_4/OMS v1.4  12/31/07/IM CN-LMLN/Saccade Enable/Enable Control/Latch2 ==
  in_1 : Inport  OutDataType=sfix(16)  OutScaling=2^0
  in_2 : Inport  Port=2  OutDataType=sfix(16)  OutScaling=2^0
  Demux : Demux  Outputs=2
  Logic : CombinatorialLogic  TruthTable=[0 1;0 1;1 0;0 1;1 0;0 1;1 0;1 0]
  Memory : Memory  Orientation=left  X0=ini
  Mux : Mux  Inputs=3
  out_1 : Outport  OutDataType=sfix(16)  OutScaling=2^0  InitialOutput=0
  out_2 : Outport  Port=2  OutDataType=sfix(16)  OutScaling=2^0  InitialOutput=0
  wires:
  in_2/1 -> Mux/3
  in_1/1 -> Mux/2
  Memory/1 -> Mux/1
  Demux/1 -> Memory/1, out_1/1
  Mux/1 -> Logic/1
  Logic/1 -> Demux/1
  Demux/2 -> out_2/1

== system OMSv1_4/OMS v1.4  12/31/07/IM CN-LMLN/Saccade Enable/Enable Control/Latch3 ==
  in_1 : Inport  OutDataType=sfix(16)  OutScaling=2^0
  in_2 : Inport  Port=2  OutDataType=sfix(16)  OutScaling=2^0
  Demux : Demux  Outputs=2
  Logic : CombinatorialLogic  TruthTable=[0 1;0 1;1 0;0 1;1 0;0 1;1 0;1 0]
  Memory : Memory  Orientation=left  X0=ini
  Mux : Mux  Inputs=3
  out_1 : Outport  OutDataType=sfix(16)  OutScaling=2^0  InitialOutput=0
  out_2 : Outport  Port=2  OutDataType=sfix(16)  OutScaling=2^0  InitialOutput=0
  wires:
  Demux/2 -> out_2/1
  Logic/1 -> Demux/1
  Mux/1 -> Logic/1
  Demux/1 -> out_1/1, Memory/1
  Memory/1 -> Mux/1
  in_1/1 -> Mux/2
  in_2/1 -> Mux/3

== system OMSv1_4/OMS v1.4  12/31/07/IM CN-LMLN/Saccade Enable/Enable Control/event timer1 ==
  note: Resettable
      | Event Timer
  note: This block is an RESETTABLE EVENT TIMER.  It outputs a spike of unit height xx milliseconds
      | (set by "timer value") after it detects an event ( i.e a TRAILING edge which represents the end of a
      |  saccadic pulse)
  note: (Init input: 0)
  note: (FF init state: Q=0)
  note: (Init input: 0)
  note: Therefore, an event first RESETS and then SETS the flip-flop.
  note: The "OR" gate allows either of these conditions to reset the circuit.  The delay before the
      | "S" input of the flip-flop prevents both "S" and "R" from being set simultaneously, because
      | this would put the flip-flop in an undefined state.
  note: The real trick here is understanding how to reload the countdown.
      | It resets if either of two conditions is met:
  note: It has TWO modes: 1) Event resettable and 2) Event Non-resettable
  note: In 1), Any event (leading or trailing edge) will reset the counter so that it
      | counts down from the end trailing edge) of that event.
  note: 1) The count reaches its limit (set in "timer value") -- Both case 1) and 2)
  note: 2) A new event (leading or trailing edge) is detected. -- Only case 1)
  note: In 2) Subsequent events DO NOT reset the counter; it only resets when it
      | reaches zero
  SW out : Inport  OutDataType=sfix(16)  OutScaling=2^0
  _timer value (port) : Inport  Port=2  OutDataType=sfix(16)  OutScaling=2^0
  1 msec : TransportDelay  DelayTime=.001
  Clock : Clock
      settings: Decimation=10
  Latch1 : Subsystem  mask(Latch){@1=0}
      mask prompts: @1 "Initial State for Output "Q":"
      mask help: Latch
      mask init:
      | ini=(@1~=0);
      mask Help: Latches the S input.  When S (set) is one, the Q output  becomes one.  The output remains one until the R (reset) input becomes one, forcing the output to zero.  If both R and S are one, the latch will be in an undefined state.
      mask Display: disp('S   Q\n\nR  !Q')
  Logical Operator : Logic  Operator=OR  Inputs=3
  Logical Operator1 : Logic
  Logical Operator2 : Logic
  Relational Operator : RelationalOperator  InputSameDT=on
  SampHold?1 : Subsystem
      mask Display: disp('S&H\n(S=L)\n(H=H)')
  Sum : Sum  Inputs=+-  OutDataType=sfix(16)  OutScaling=2^0  SaturateOnIntegerOverflow=on  InputSameDT=on
  Terminator : Terminator
  event resettable? : Constant  Orientation=up  OutDataType=sfix(16)  OutScaling=2^0
  leading edge detect : Subsystem
      mask Display: disp('Leading\nEdge Det')
  loop breaker : Memory  Orientation=left
  trailing edge detect : Subsystem
      mask Display: disp('Trailing\nEdge Det')
  FF Reset : Outport  OutDataType=sfix(16)  OutScaling=2^0  InitialOutput=0
  wires:
  _timer value (port)/1 -> Relational Operator/2
  1 msec/1 -> Latch1/1(in_1)
  Logical Operator/1 -> Latch1/2(in_2)
  SampHold?1/1(output) -> Sum/2
  Relational Operator/1 -> loop breaker/1, FF Reset/1
  SW out/1 -> trailing edge detect/1(in_1), leading edge detect/1(in_1)
  Clock/1 -> Sum/1, SampHold?1/1(Input)
  Sum/1 -> Relational Operator/1
  Latch1/1(out_1) -> SampHold?1/2(S/H?)
  loop breaker/1 -> Logical Operator/3
  Logical Operator1/1 -> Logical Operator/1
  trailing edge detect/1(out_1) -> Logical Operator1/1, 1 msec/1
  Logical Operator2/1 -> Logical Operator/2
  leading edge detect/1(out_1) -> Logical Operator2/1
  event resettable?/1 -> Logical Operator2/2, Logical Operator1/2
  Latch1/2(out_2) -> Terminator/1

== system OMSv1_4/OMS v1.4  12/31/07/IM CN-LMLN/Saccade Enable/Enable Control/leading edge detect ==
  note: It is also possible to remove the SIGNUM function
      | and the '==', and replace them with a simple
      | switch with a threshold of (say) 150 or so.
  note: leading edge detection
  in_1 : Inport  OutDataType=sfix(16)  OutScaling=2^0
  Abs : Abs  SaturateOnIntegerOverflow=on
  Derivative : Derivative
  Relational Operator : RelationalOperator  Operator===  InputSameDT=on
  Sign : Subsystem
      mask Type: Sign
      mask Description: y = sign(x)
      mask Help: Sign Function:\n\t\t\ty = 1 if x > 0\n\t\t\ty = 0 if x = 0\n\t\t\ty = -1 if x < 0
      mask Display: plot(-50,-50,50,50,[-50,50],[0,0],[0,0],[-50,50],[-40,0],[-30,-30],[0,40],[30,30])
  Threshold 1 : Constant  OutDataType=sfix(16)  OutScaling=2^0
  out_1 : Outport  OutDataType=sfix(16)  OutScaling=2^0  InitialOutput=0
  wires:
  Abs/1 -> Derivative/1
  Derivative/1 -> Sign/1(in_1)
  Sign/1(out_1) -> Relational Operator/1
  Threshold 1/1 -> Relational Operator/2
  Relational Operator/1 -> out_1/1
  in_1/1 -> Abs/1

== system OMSv1_4/OMS v1.4  12/31/07/IM CN-LMLN/Saccade Enable/Enable Control/leading edge detect2 ==
  note: leading edge detection
  note: It is also possible to remove the SIGNUM function
      | and the '==', and replace them with a simple
      | switch with a threshold of (say) 150 or so.
  in_1 : Inport  OutDataType=sfix(16)  OutScaling=2^0
  Abs : Abs  SaturateOnIntegerOverflow=on
  Derivative : Derivative
  Relational Operator : RelationalOperator  Operator===  InputSameDT=on
  Sign : Subsystem
      mask Type: Sign
      mask Description: y = sign(x)
      mask Help: Sign Function:\n\t\t\ty = 1 if x > 0\n\t\t\ty = 0 if x = 0\n\t\t\ty = -1 if x < 0
      mask Display: plot(-50,-50,50,50,[-50,50],[0,0],[0,0],[-50,50],[-40,0],[-30,-30],[0,40],[30,30])
  Threshold 1 : Constant  OutDataType=sfix(16)  OutScaling=2^0
  out_1 : Outport  OutDataType=sfix(16)  OutScaling=2^0  InitialOutput=0
  wires:
  in_1/1 -> Abs/1
  Relational Operator/1 -> out_1/1
  Threshold 1/1 -> Relational Operator/2
  Sign/1(out_1) -> Relational Operator/1
  Derivative/1 -> Sign/1(in_1)
  Abs/1 -> Derivative/1

== system OMSv1_4/OMS v1.4  12/31/07/IM CN-LMLN/Saccade Enable/Enable Control/trailing edge detect ==
  note: It is also possible to remove the SIGNUM function
      | and the '==', and replace them with a simple
      | switch with a threshold of (say) 150 or so.
  note: trailing edge detection
  PG : Inport  OutDataType=sfix(16)  OutScaling=2^0
  Abs : Abs  SaturateOnIntegerOverflow=on
  Derivative : Derivative
  Relational Operator : RelationalOperator  Operator===  InputSameDT=on
  Sign : Subsystem
      mask Type: Sign
      mask Description: y = sign(x)
      mask Help: Sign Function:\n\t\t\ty = 1 if x > 0\n\t\t\ty = 0 if x = 0\n\t\t\ty = -1 if x < 0
      mask Display: plot(-50,-50,50,50,[-50,50],[0,0],[0,0],[-50,50],[-40,0],[-30,-30],[0,40],[30,30])
  Threshold 1 : Constant  Value=-1  OutDataType=sfix(16)  OutScaling=2^0
  Latch R : Outport  OutDataType=sfix(16)  OutScaling=2^0  InitialOutput=0
  wires:
  Abs/1 -> Derivative/1
  Derivative/1 -> Sign/1(in_1)
  Sign/1(out_1) -> Relational Operator/1
  Threshold 1/1 -> Relational Operator/2
  Relational Operator/1 -> Latch R/1
  PG/1 -> Abs/1

== system OMSv1_4/OMS v1.4  12/31/07/IM CN-LMLN/Saccade Enable/LN FPh Gen/DZ 4 ==
  note: This block is a better implementation of a dead zone than  the
      | block supplied by SIMULINK, because here we don't _subtract_
      | the dead zone from the rest of output.
  note: We just output zero when the dead zone is in effect, and leave the
      |  output alone the rest of the time.
  in_1 : Inport  OutDataType=sfix(16)  OutScaling=2^0
  Abs : Abs  Orientation=down  SaturateOnIntegerOverflow=on
  Relational Operator : RelationalOperator  InputSameDT=on
  Switch6 : Switch  Threshold=.5  SaturateOnIntegerOverflow=on  InputSameDT=on
  dead zone : Constant  Orientation=up  Value=4  OutDataType=sfix(16)  OutScaling=2^0
  pos (deg) criterion1 : Constant  Orientation=left  Value=0  OutDataType=sfix(16)  OutScaling=2^0
  out_1 : Outport  OutDataType=sfix(16)  OutScaling=2^0  InitialOutput=0
  wires:
  Switch6/1 -> out_1/1
  in_1/1 -> Switch6/1, Abs/1
  Abs/1 -> Relational Operator/1
  pos (deg) criterion1/1 -> Switch6/3
  dead zone/1 -> Relational Operator/2
  Relational Operator/1 -> Switch6/2
